simulink model "Electrical_System_2018b_obfs"  (R2019b)
settings: Solver=VariableStepAuto  StartTime=0.0  StopTime=5  RelTol=1e-3  AbsTol=1e-3  EnableMultiTasking=on
InitFcn:
  | Steady_State_Initialisation;
StopFcn:
  | %sscexplore(simlog);
  | %Logging
undefined symbols (not defined in the file): abrlhklxvp, aexgmhuedq, afmfmjnutg, afpphrjpnc, ahuxbyvruc, alarvljztt, amxnyqmnuw, aodrlwvqie, aolhmuplyq, aqpmguuqkg, auesgwirzl, aurophlnng, awamelrhru, ayfhvxflxn, azxkacuhqc, babszerikg, bawhdqanwq, bevoqecvei, bltjvqbchx, bmqsuewujl, bsmyqjfgnf, btvjbsmnve, bywgxqeadw, bziaduxaer, bzmcmdqocb, bzsvyvetat, ccsjnrbsih, cdvenygxwh, cedkrnslhx, cjheorclzs, cjrdshrtqx, ckhavyhcza, ckxewznhlz, cmrcgyiplk, conenicnws, cqkejbgjnn, csfnuwymhe, cunupkhwbh, cwzfvzuxxh, dcadmadufn, dcfponivnv, ddtrqjrhjn, dfhoxvkqas, dfrhtcwpne, dfvomcagjv, djijwylxea, dnmeqksrrm, dnzewbdkaa, dsqcykyxav, dtswwlttmm, ecumpidjtv, edegaywrct, ejjjsmnejc, eknqnehjdz, emvdetzouf, esxbqkbahr, etnkkbreiq, eunoiiiirw, ewewcuedir, fatkfxdhtc ... (+386)
libraries: fl_lib x802, ee_lib x362, fl_ps_legacy_lib x160, nesl_utility x85
(part 26 of 26)

== system Electrical_System_2018b_obfs/Redacted_1221/Redacted_7996/Redacted_7418/Redacted_4377/Redacted_6082/Redacted_3086/Redacted_7741 ==
  Redacted_4240 : fl_lib/Electrical/Electrical Elements/Open Circuit  v_specify=off  v_priority=None  v=ebhsjuvrvm V  v_nominal_specify=off  v_nominal_unit=V  v_nominal_value=uogdcjcffr
      settings: SourceProductName=Simscape  SourceProductBaseCode=SS
  Redacted_6054 : PMIOPort  Side=Left
  Redacted_5626 : PMIOPort  Port=2  Side=Left
  Redacted_6271 : PMIOPort  Port=3  Side=Left
  Redacted_2564 : PMIOPort  Port=4  Side=Right
  Redacted_7933 : PMIOPort  Port=5  Side=Right
  connections:
  Redacted_4240/LConn1 -- Redacted_5626/RConn1
  Redacted_2564/RConn1 -- Redacted_6054/RConn1
  Redacted_7933/RConn1 -- Redacted_6271/RConn1

== system Electrical_System_2018b_obfs/Redacted_1221/Redacted_7996/Redacted_7418/Redacted_4377/Redacted_6082/Redacted_3818/Neutral_Negative ==
  Open Circuit : fl_lib/Electrical/Electrical Elements/Open Circuit  v_specify=off  v_priority=None  v=0 V  v_nominal_specify=off  v_nominal_unit=V  v_nominal_value=1
      settings: SourceProductName=Simscape  SourceProductBaseCode=SS
  Redacted_558 : PMIOPort  Side=Left
  Redacted_9353 : PMIOPort  Port=2  Side=Left
  Redacted_2763 : PMIOPort  Port=3  Side=Left
  Redacted_5509 : PMIOPort  Port=4  Side=Right
  Redacted_3127 : PMIOPort  Port=5  Side=Right
  connections:
  Redacted_9353/RConn1 -- Redacted_5509/RConn1
  Open Circuit/LConn1 -- Redacted_558/RConn1
  Redacted_3127/RConn1 -- Redacted_2763/RConn1

== system Electrical_System_2018b_obfs/Redacted_1221/Redacted_7996/Redacted_7418/Redacted_4377/Redacted_6082/Redacted_3818/Positive_Neutral ==
  Open Circuit : fl_lib/Electrical/Electrical Elements/Open Circuit  v_specify=off  v_priority=None  v=0 V  v_nominal_specify=off  v_nominal_unit=V  v_nominal_value=1
      settings: SourceProductName=Simscape  SourceProductBaseCode=SS
  Redacted_558 : PMIOPort  Side=Left
  Redacted_9353 : PMIOPort  Port=2  Side=Left
  Redacted_2763 : PMIOPort  Port=3  Side=Left
  Redacted_5509 : PMIOPort  Port=4  Side=Right
  Redacted_3127 : PMIOPort  Port=5  Side=Right
  connections:
  Redacted_9353/RConn1 -- Redacted_3127/RConn1
  Redacted_5509/RConn1 -- Redacted_558/RConn1
  Open Circuit/LConn1 -- Redacted_2763/RConn1

== system Electrical_System_2018b_obfs/Redacted_1221/Redacted_7996/Redacted_7418/Redacted_4377/Redacted_6082/Redacted_3818/Redacted_7647 ==
  Redacted_9625 : fl_lib/Electrical/Electrical Elements/Open Circuit  v_specify=off  v_priority=None  v=ubfstcorvt V  v_nominal_specify=off  v_nominal_unit=V  v_nominal_value=abvsahtgbf
      settings: SourceProductName=Simscape  SourceProductBaseCode=SS
  Redacted_558 : PMIOPort  Side=Left
  Redacted_9353 : PMIOPort  Port=2  Side=Left
  Redacted_2763 : PMIOPort  Port=3  Side=Left
  Redacted_5509 : PMIOPort  Port=4  Side=Right
  Redacted_3127 : PMIOPort  Port=5  Side=Right
  connections:
  Redacted_3127/RConn1 -- Redacted_2763/RConn1
  Redacted_5509/RConn1 -- Redacted_558/RConn1
  Redacted_9625/LConn1 -- Redacted_9353/RConn1

== system Electrical_System_2018b_obfs/Redacted_1221/Redacted_7996/Redacted_7418/Redacted_4377/Redacted_6082/Redacted_4174/Neutral_Negative ==
  Open Circuit : fl_lib/Electrical/Electrical Elements/Open Circuit  v_specify=off  v_priority=None  v=0 V  v_nominal_specify=off  v_nominal_unit=V  v_nominal_value=1
      settings: SourceProductName=Simscape  SourceProductBaseCode=SS
  Redacted_9679 : PMIOPort  Side=Left
  Redacted_9878 : PMIOPort  Port=2  Side=Left
  Redacted_224 : PMIOPort  Port=3  Side=Left
  Redacted_5953 : PMIOPort  Port=4  Side=Right
  Redacted_7639 : PMIOPort  Port=5  Side=Right
  connections:
  Redacted_9878/RConn1 -- Redacted_5953/RConn1
  Open Circuit/LConn1 -- Redacted_9679/RConn1
  Redacted_7639/RConn1 -- Redacted_224/RConn1

== system Electrical_System_2018b_obfs/Redacted_1221/Redacted_7996/Redacted_7418/Redacted_4377/Redacted_6082/Redacted_4174/Positive_Neutral ==
  Open Circuit : fl_lib/Electrical/Electrical Elements/Open Circuit  v_specify=off  v_priority=None  v=0 V  v_nominal_specify=off  v_nominal_unit=V  v_nominal_value=1
      settings: SourceProductName=Simscape  SourceProductBaseCode=SS
  Redacted_9679 : PMIOPort  Side=Left
  Redacted_9878 : PMIOPort  Port=2  Side=Left
  Redacted_224 : PMIOPort  Port=3  Side=Left
  Redacted_5953 : PMIOPort  Port=4  Side=Right
  Redacted_7639 : PMIOPort  Port=5  Side=Right
  connections:
  Redacted_9878/RConn1 -- Redacted_7639/RConn1
  Redacted_5953/RConn1 -- Redacted_9679/RConn1
  Open Circuit/LConn1 -- Redacted_224/RConn1

== system Electrical_System_2018b_obfs/Redacted_1221/Redacted_7996/Redacted_7418/Redacted_4377/Redacted_6082/Redacted_4174/Redacted_8370 ==
  Redacted_7682 : fl_lib/Electrical/Electrical Elements/Open Circuit  v_specify=off  v_priority=None  v=krmygfnnpy V  v_nominal_specify=off  v_nominal_unit=V  v_nominal_value=lqikwmhyvq
      settings: SourceProductName=Simscape  SourceProductBaseCode=SS
  Redacted_9679 : PMIOPort  Side=Left
  Redacted_9878 : PMIOPort  Port=2  Side=Left
  Redacted_224 : PMIOPort  Port=3  Side=Left
  Redacted_5953 : PMIOPort  Port=4  Side=Right
  Redacted_7639 : PMIOPort  Port=5  Side=Right
  connections:
  Redacted_7639/RConn1 -- Redacted_224/RConn1
  Redacted_5953/RConn1 -- Redacted_9679/RConn1
  Redacted_7682/LConn1 -- Redacted_9878/RConn1

== system Electrical_System_2018b_obfs/Redacted_1221/Redacted_7996/Redacted_7418/Redacted_4377/Redacted_6082/Redacted_4278/Neutral_Negative ==
  Open Circuit : fl_lib/Electrical/Electrical Elements/Open Circuit  v_specify=off  v_priority=None  v=0 V  v_nominal_specify=off  v_nominal_unit=V  v_nominal_value=1
      settings: SourceProductName=Simscape  SourceProductBaseCode=SS
  Redacted_1495 : PMIOPort  Side=Left
  Redacted_2064 : PMIOPort  Port=2  Side=Left
  Redacted_9467 : PMIOPort  Port=3  Side=Left
  Redacted_1543 : PMIOPort  Port=4  Side=Right
  Redacted_9491 : PMIOPort  Port=5  Side=Right
  connections:
  Redacted_9491/RConn1 -- Redacted_9467/RConn1
  Open Circuit/LConn1 -- Redacted_1495/RConn1
  Redacted_2064/RConn1 -- Redacted_1543/RConn1

== system Electrical_System_2018b_obfs/Redacted_1221/Redacted_7996/Redacted_7418/Redacted_4377/Redacted_6082/Redacted_4278/Positive_Neutral ==
  Open Circuit : fl_lib/Electrical/Electrical Elements/Open Circuit  v_specify=off  v_priority=None  v=0 V  v_nominal_specify=off  v_nominal_unit=V  v_nominal_value=1
      settings: SourceProductName=Simscape  SourceProductBaseCode=SS
  Redacted_1495 : PMIOPort  Side=Left
  Redacted_2064 : PMIOPort  Port=2  Side=Left
  Redacted_9467 : PMIOPort  Port=3  Side=Left
  Redacted_1543 : PMIOPort  Port=4  Side=Right
  Redacted_9491 : PMIOPort  Port=5  Side=Right
  connections:
  Open Circuit/LConn1 -- Redacted_9467/RConn1
  Redacted_1543/RConn1 -- Redacted_1495/RConn1
  Redacted_2064/RConn1 -- Redacted_9491/RConn1

== system Electrical_System_2018b_obfs/Redacted_1221/Redacted_7996/Redacted_7418/Redacted_4377/Redacted_6082/Redacted_4278/Redacted_1592 ==
  Redacted_6518 : fl_lib/Electrical/Electrical Elements/Open Circuit  v_specify=off  v_priority=None  v=kniygukgpp V  v_nominal_specify=off  v_nominal_unit=V  v_nominal_value=dzkrotrooy
      settings: SourceProductName=Simscape  SourceProductBaseCode=SS
  Redacted_1495 : PMIOPort  Side=Left
  Redacted_2064 : PMIOPort  Port=2  Side=Left
  Redacted_9467 : PMIOPort  Port=3  Side=Left
  Redacted_1543 : PMIOPort  Port=4  Side=Right
  Redacted_9491 : PMIOPort  Port=5  Side=Right
  connections:
  Redacted_6518/LConn1 -- Redacted_2064/RConn1
  Redacted_1543/RConn1 -- Redacted_1495/RConn1
  Redacted_9491/RConn1 -- Redacted_9467/RConn1

== system Electrical_System_2018b_obfs/Redacted_1221/Redacted_7996/Redacted_7418/Redacted_4377/Redacted_6082/Redacted_4413/Neutral_Negative ==
  Open Circuit : fl_lib/Electrical/Electrical Elements/Open Circuit  v_specify=off  v_priority=None  v=0 V  v_nominal_specify=off  v_nominal_unit=V  v_nominal_value=1
      settings: SourceProductName=Simscape  SourceProductBaseCode=SS
  Redacted_9976 : PMIOPort  Side=Left
  Redacted_5180 : PMIOPort  Port=2  Side=Left
  Redacted_6712 : PMIOPort  Port=3  Side=Left
  Redacted_6595 : PMIOPort  Port=4  Side=Right
  Redacted_8408 : PMIOPort  Port=5  Side=Right
  connections:
  Redacted_8408/RConn1 -- Redacted_6712/RConn1
  Open Circuit/LConn1 -- Redacted_9976/RConn1
  Redacted_5180/RConn1 -- Redacted_6595/RConn1

== system Electrical_System_2018b_obfs/Redacted_1221/Redacted_7996/Redacted_7418/Redacted_4377/Redacted_6082/Redacted_4413/Positive_Neutral ==
  Open Circuit : fl_lib/Electrical/Electrical Elements/Open Circuit  v_specify=off  v_priority=None  v=0 V  v_nominal_specify=off  v_nominal_unit=V  v_nominal_value=1
      settings: SourceProductName=Simscape  SourceProductBaseCode=SS
  Redacted_9976 : PMIOPort  Side=Left
  Redacted_5180 : PMIOPort  Port=2  Side=Left
  Redacted_6712 : PMIOPort  Port=3  Side=Left
  Redacted_6595 : PMIOPort  Port=4  Side=Right
  Redacted_8408 : PMIOPort  Port=5  Side=Right
  connections:
  Open Circuit/LConn1 -- Redacted_6712/RConn1
  Redacted_6595/RConn1 -- Redacted_9976/RConn1
  Redacted_5180/RConn1 -- Redacted_8408/RConn1

== system Electrical_System_2018b_obfs/Redacted_1221/Redacted_7996/Redacted_7418/Redacted_4377/Redacted_6082/Redacted_4413/Redacted_6190 ==
  Redacted_6825 : fl_lib/Electrical/Electrical Elements/Open Circuit  v_specify=off  v_priority=None  v=nafaxblafc V  v_nominal_specify=off  v_nominal_unit=V  v_nominal_value=uctqgjleyg
      settings: SourceProductName=Simscape  SourceProductBaseCode=SS
  Redacted_9976 : PMIOPort  Side=Left
  Redacted_5180 : PMIOPort  Port=2  Side=Left
  Redacted_6712 : PMIOPort  Port=3  Side=Left
  Redacted_6595 : PMIOPort  Port=4  Side=Right
  Redacted_8408 : PMIOPort  Port=5  Side=Right
  connections:
  Redacted_6825/LConn1 -- Redacted_5180/RConn1
  Redacted_6595/RConn1 -- Redacted_9976/RConn1
  Redacted_8408/RConn1 -- Redacted_6712/RConn1

== system Electrical_System_2018b_obfs/Redacted_1221/Redacted_7996/Redacted_7418/Redacted_4377/Redacted_6082/Redacted_5550/Neutral_Negative ==
  Open Circuit : fl_lib/Electrical/Electrical Elements/Open Circuit  v_specify=off  v_priority=None  v=0 V  v_nominal_specify=off  v_nominal_unit=V  v_nominal_value=1
      settings: SourceProductName=Simscape  SourceProductBaseCode=SS
  Redacted_6826 : PMIOPort  Side=Left
  Redacted_51 : PMIOPort  Port=2  Side=Left
  Redacted_9515 : PMIOPort  Port=3  Side=Left
  Redacted_375 : PMIOPort  Port=4  Side=Right
  Redacted_6304 : PMIOPort  Port=5  Side=Right
  connections:
  Redacted_6304/RConn1 -- Redacted_9515/RConn1
  Open Circuit/LConn1 -- Redacted_6826/RConn1
  Redacted_51/RConn1 -- Redacted_375/RConn1

== system Electrical_System_2018b_obfs/Redacted_1221/Redacted_7996/Redacted_7418/Redacted_4377/Redacted_6082/Redacted_5550/Positive_Neutral ==
  Open Circuit : fl_lib/Electrical/Electrical Elements/Open Circuit  v_specify=off  v_priority=None  v=0 V  v_nominal_specify=off  v_nominal_unit=V  v_nominal_value=1
      settings: SourceProductName=Simscape  SourceProductBaseCode=SS
  Redacted_6826 : PMIOPort  Side=Left
  Redacted_51 : PMIOPort  Port=2  Side=Left
  Redacted_9515 : PMIOPort  Port=3  Side=Left
  Redacted_375 : PMIOPort  Port=4  Side=Right
  Redacted_6304 : PMIOPort  Port=5  Side=Right
  connections:
  Open Circuit/LConn1 -- Redacted_9515/RConn1
  Redacted_375/RConn1 -- Redacted_6826/RConn1
  Redacted_51/RConn1 -- Redacted_6304/RConn1

== system Electrical_System_2018b_obfs/Redacted_1221/Redacted_7996/Redacted_7418/Redacted_4377/Redacted_6082/Redacted_5550/Redacted_2952 ==
  Redacted_9904 : fl_lib/Electrical/Electrical Elements/Open Circuit  v_specify=off  v_priority=None  v=cbwtykvznf V  v_nominal_specify=off  v_nominal_unit=V  v_nominal_value=bbwdbtprkb
      settings: SourceProductName=Simscape  SourceProductBaseCode=SS
  Redacted_6826 : PMIOPort  Side=Left
  Redacted_51 : PMIOPort  Port=2  Side=Left
  Redacted_9515 : PMIOPort  Port=3  Side=Left
  Redacted_375 : PMIOPort  Port=4  Side=Right
  Redacted_6304 : PMIOPort  Port=5  Side=Right
  connections:
  Redacted_9904/LConn1 -- Redacted_51/RConn1
  Redacted_375/RConn1 -- Redacted_6826/RConn1
  Redacted_6304/RConn1 -- Redacted_9515/RConn1

== system Electrical_System_2018b_obfs/Redacted_1221/Redacted_7996/Redacted_7418/Redacted_4377/Redacted_6082/Redacted_5713/Neutral_Negative ==
  Open Circuit : fl_lib/Electrical/Electrical Elements/Open Circuit  v_specify=off  v_priority=None  v=0 V  v_nominal_specify=off  v_nominal_unit=V  v_nominal_value=1
      settings: SourceProductName=Simscape  SourceProductBaseCode=SS
  Redacted_6138 : PMIOPort  Side=Left
  Redacted_1431 : PMIOPort  Port=2  Side=Left
  Redacted_7946 : PMIOPort  Port=3  Side=Left
  Redacted_819 : PMIOPort  Port=4  Side=Right
  Redacted_4816 : PMIOPort  Port=5  Side=Right
  connections:
  Redacted_4816/RConn1 -- Redacted_7946/RConn1
  Open Circuit/LConn1 -- Redacted_6138/RConn1
  Redacted_1431/RConn1 -- Redacted_819/RConn1

== system Electrical_System_2018b_obfs/Redacted_1221/Redacted_7996/Redacted_7418/Redacted_4377/Redacted_6082/Redacted_5713/Positive_Neutral ==
  Open Circuit : fl_lib/Electrical/Electrical Elements/Open Circuit  v_specify=off  v_priority=None  v=0 V  v_nominal_specify=off  v_nominal_unit=V  v_nominal_value=1
      settings: SourceProductName=Simscape  SourceProductBaseCode=SS
  Redacted_6138 : PMIOPort  Side=Left
  Redacted_1431 : PMIOPort  Port=2  Side=Left
  Redacted_7946 : PMIOPort  Port=3  Side=Left
  Redacted_819 : PMIOPort  Port=4  Side=Right
  Redacted_4816 : PMIOPort  Port=5  Side=Right
  connections:
  Open Circuit/LConn1 -- Redacted_7946/RConn1
  Redacted_819/RConn1 -- Redacted_6138/RConn1
  Redacted_1431/RConn1 -- Redacted_4816/RConn1

== system Electrical_System_2018b_obfs/Redacted_1221/Redacted_7996/Redacted_7418/Redacted_4377/Redacted_6082/Redacted_5713/Redacted_1184 ==
  Redacted_2299 : fl_lib/Electrical/Electrical Elements/Open Circuit  v_specify=off  v_priority=None  v=tqpmitufxi V  v_nominal_specify=off  v_nominal_unit=V  v_nominal_value=nizvadugds
      settings: SourceProductName=Simscape  SourceProductBaseCode=SS
  Redacted_6138 : PMIOPort  Side=Left
  Redacted_1431 : PMIOPort  Port=2  Side=Left
  Redacted_7946 : PMIOPort  Port=3  Side=Left
  Redacted_819 : PMIOPort  Port=4  Side=Right
  Redacted_4816 : PMIOPort  Port=5  Side=Right
  connections:
  Redacted_2299/LConn1 -- Redacted_1431/RConn1
  Redacted_819/RConn1 -- Redacted_6138/RConn1
  Redacted_4816/RConn1 -- Redacted_7946/RConn1

== system Electrical_System_2018b_obfs/Redacted_1221/Redacted_7996/Redacted_7418/Redacted_4377/Redacted_6082/Redacted_5976/Neutral_Negative ==
  Open Circuit : fl_lib/Electrical/Electrical Elements/Open Circuit  v_specify=off  v_priority=None  v=0 V  v_nominal_specify=off  v_nominal_unit=V  v_nominal_value=1
      settings: SourceProductName=Simscape  SourceProductBaseCode=SS
  Redacted_9241 : PMIOPort  Side=Left
  Redacted_5276 : PMIOPort  Port=2  Side=Left
  Redacted_2400 : PMIOPort  Port=3  Side=Left
  Redacted_5406 : PMIOPort  Port=4  Side=Right
  Redacted_1074 : PMIOPort  Port=5  Side=Right
  connections:
  Redacted_5276/RConn1 -- Redacted_5406/RConn1
  Open Circuit/LConn1 -- Redacted_9241/RConn1
  Redacted_1074/RConn1 -- Redacted_2400/RConn1

== system Electrical_System_2018b_obfs/Redacted_1221/Redacted_7996/Redacted_7418/Redacted_4377/Redacted_6082/Redacted_5976/Positive_Neutral ==
  Open Circuit : fl_lib/Electrical/Electrical Elements/Open Circuit  v_specify=off  v_priority=None  v=0 V  v_nominal_specify=off  v_nominal_unit=V  v_nominal_value=1
      settings: SourceProductName=Simscape  SourceProductBaseCode=SS
  Redacted_9241 : PMIOPort  Side=Left
  Redacted_5276 : PMIOPort  Port=2  Side=Left
  Redacted_2400 : PMIOPort  Port=3  Side=Left
  Redacted_5406 : PMIOPort  Port=4  Side=Right
  Redacted_1074 : PMIOPort  Port=5  Side=Right
  connections:
  Redacted_5276/RConn1 -- Redacted_1074/RConn1
  Redacted_5406/RConn1 -- Redacted_9241/RConn1
  Open Circuit/LConn1 -- Redacted_2400/RConn1

== system Electrical_System_2018b_obfs/Redacted_1221/Redacted_7996/Redacted_7418/Redacted_4377/Redacted_6082/Redacted_5976/Redacted_5620 ==
  Redacted_9178 : fl_lib/Electrical/Electrical Elements/Open Circuit  v_specify=off  v_priority=None  v=jhtpowznxh V  v_nominal_specify=off  v_nominal_unit=V  v_nominal_value=mubuuhzqmu
      settings: SourceProductName=Simscape  SourceProductBaseCode=SS
  Redacted_9241 : PMIOPort  Side=Left
  Redacted_5276 : PMIOPort  Port=2  Side=Left
  Redacted_2400 : PMIOPort  Port=3  Side=Left
  Redacted_5406 : PMIOPort  Port=4  Side=Right
  Redacted_1074 : PMIOPort  Port=5  Side=Right
  connections:
  Redacted_1074/RConn1 -- Redacted_2400/RConn1
  Redacted_5406/RConn1 -- Redacted_9241/RConn1
  Redacted_9178/LConn1 -- Redacted_5276/RConn1

== system Electrical_System_2018b_obfs/Redacted_1221/Redacted_7996/Redacted_7418/Redacted_4377/Redacted_6082/Redacted_6424/Neutral_Negative ==
  Open Circuit : fl_lib/Electrical/Electrical Elements/Open Circuit  v_specify=off  v_priority=None  v=0 V  v_nominal_specify=off  v_nominal_unit=V  v_nominal_value=1
      settings: SourceProductName=Simscape  SourceProductBaseCode=SS
  Redacted_4582 : PMIOPort  Side=Left
  Redacted_1544 : PMIOPort  Port=2  Side=Left
  Redacted_1581 : PMIOPort  Port=3  Side=Left
  Redacted_1961 : PMIOPort  Port=4  Side=Right
  Redacted_7479 : PMIOPort  Port=5  Side=Right
  connections:
  Redacted_7479/RConn1 -- Redacted_1581/RConn1
  Open Circuit/LConn1 -- Redacted_4582/RConn1
  Redacted_1544/RConn1 -- Redacted_1961/RConn1

== system Electrical_System_2018b_obfs/Redacted_1221/Redacted_7996/Redacted_7418/Redacted_4377/Redacted_6082/Redacted_6424/Positive_Neutral ==
  Open Circuit : fl_lib/Electrical/Electrical Elements/Open Circuit  v_specify=off  v_priority=None  v=0 V  v_nominal_specify=off  v_nominal_unit=V  v_nominal_value=1
      settings: SourceProductName=Simscape  SourceProductBaseCode=SS
  Redacted_4582 : PMIOPort  Side=Left
  Redacted_1544 : PMIOPort  Port=2  Side=Left
  Redacted_1581 : PMIOPort  Port=3  Side=Left
  Redacted_1961 : PMIOPort  Port=4  Side=Right
  Redacted_7479 : PMIOPort  Port=5  Side=Right
  connections:
  Open Circuit/LConn1 -- Redacted_1581/RConn1
  Redacted_1961/RConn1 -- Redacted_4582/RConn1
  Redacted_1544/RConn1 -- Redacted_7479/RConn1

== system Electrical_System_2018b_obfs/Redacted_1221/Redacted_7996/Redacted_7418/Redacted_4377/Redacted_6082/Redacted_6424/Redacted_7805 ==
  Redacted_3936 : fl_lib/Electrical/Electrical Elements/Open Circuit  v_specify=off  v_priority=None  v=fjoxglgvhp V  v_nominal_specify=off  v_nominal_unit=V  v_nominal_value=omyuclhrqc
      settings: SourceProductName=Simscape  SourceProductBaseCode=SS
  Redacted_4582 : PMIOPort  Side=Left
  Redacted_1544 : PMIOPort  Port=2  Side=Left
  Redacted_1581 : PMIOPort  Port=3  Side=Left
  Redacted_1961 : PMIOPort  Port=4  Side=Right
  Redacted_7479 : PMIOPort  Port=5  Side=Right
  connections:
  Redacted_3936/LConn1 -- Redacted_1544/RConn1
  Redacted_1961/RConn1 -- Redacted_4582/RConn1
  Redacted_7479/RConn1 -- Redacted_1581/RConn1

== system Electrical_System_2018b_obfs/Redacted_1221/Redacted_7996/Redacted_7418/Redacted_4377/Redacted_6082/Redacted_7051/Neutral_Negative ==
  Open Circuit : fl_lib/Electrical/Electrical Elements/Open Circuit  v_specify=off  v_priority=None  v=0 V  v_nominal_specify=off  v_nominal_unit=V  v_nominal_value=1
      settings: SourceProductName=Simscape  SourceProductBaseCode=SS
  Redacted_2697 : PMIOPort  Side=Left
  Redacted_1518 : PMIOPort  Port=2  Side=Left
  Redacted_2395 : PMIOPort  Port=3  Side=Left
  Redacted_3537 : PMIOPort  Port=4  Side=Right
  Redacted_8383 : PMIOPort  Port=5  Side=Right
  connections:
  Redacted_1518/RConn1 -- Redacted_3537/RConn1
  Open Circuit/LConn1 -- Redacted_2697/RConn1
  Redacted_8383/RConn1 -- Redacted_2395/RConn1

== system Electrical_System_2018b_obfs/Redacted_1221/Redacted_7996/Redacted_7418/Redacted_4377/Redacted_6082/Redacted_7051/Positive_Neutral ==
  Open Circuit : fl_lib/Electrical/Electrical Elements/Open Circuit  v_specify=off  v_priority=None  v=0 V  v_nominal_specify=off  v_nominal_unit=V  v_nominal_value=1
      settings: SourceProductName=Simscape  SourceProductBaseCode=SS
  Redacted_2697 : PMIOPort  Side=Left
  Redacted_1518 : PMIOPort  Port=2  Side=Left
  Redacted_2395 : PMIOPort  Port=3  Side=Left
  Redacted_3537 : PMIOPort  Port=4  Side=Right
  Redacted_8383 : PMIOPort  Port=5  Side=Right
  connections:
  Redacted_1518/RConn1 -- Redacted_8383/RConn1
  Redacted_3537/RConn1 -- Redacted_2697/RConn1
  Open Circuit/LConn1 -- Redacted_2395/RConn1

== system Electrical_System_2018b_obfs/Redacted_1221/Redacted_7996/Redacted_7418/Redacted_4377/Redacted_6082/Redacted_7051/Redacted_1021 ==
  Redacted_3666 : fl_lib/Electrical/Electrical Elements/Open Circuit  v_specify=off  v_priority=None  v=jitpzdpdri V  v_nominal_specify=off  v_nominal_unit=V  v_nominal_value=zhywmqlonq
      settings: SourceProductName=Simscape  SourceProductBaseCode=SS
  Redacted_2697 : PMIOPort  Side=Left
  Redacted_1518 : PMIOPort  Port=2  Side=Left
  Redacted_2395 : PMIOPort  Port=3  Side=Left
  Redacted_3537 : PMIOPort  Port=4  Side=Right
  Redacted_8383 : PMIOPort  Port=5  Side=Right
  connections:
  Redacted_8383/RConn1 -- Redacted_2395/RConn1
  Redacted_3537/RConn1 -- Redacted_2697/RConn1
  Redacted_3666/LConn1 -- Redacted_1518/RConn1

== system Electrical_System_2018b_obfs/Redacted_1221/Redacted_7996/Redacted_7418/Redacted_4377/Redacted_6082/Redacted_7884/Neutral_Negative ==
  Open Circuit : fl_lib/Electrical/Electrical Elements/Open Circuit  v_specify=off  v_priority=None  v=0 V  v_nominal_specify=off  v_nominal_unit=V  v_nominal_value=1
      settings: SourceProductName=Simscape  SourceProductBaseCode=SS
  Redacted_6224 : PMIOPort  Side=Left
  Redacted_4321 : PMIOPort  Port=2  Side=Left
  Redacted_2243 : PMIOPort  Port=3  Side=Left
  Redacted_707 : PMIOPort  Port=4  Side=Right
  Redacted_8636 : PMIOPort  Port=5  Side=Right
  connections:
  Redacted_4321/RConn1 -- Redacted_707/RConn1
  Open Circuit/LConn1 -- Redacted_6224/RConn1
  Redacted_8636/RConn1 -- Redacted_2243/RConn1

== system Electrical_System_2018b_obfs/Redacted_1221/Redacted_7996/Redacted_7418/Redacted_4377/Redacted_6082/Redacted_7884/Positive_Neutral ==
  Open Circuit : fl_lib/Electrical/Electrical Elements/Open Circuit  v_specify=off  v_priority=None  v=0 V  v_nominal_specify=off  v_nominal_unit=V  v_nominal_value=1
      settings: SourceProductName=Simscape  SourceProductBaseCode=SS
  Redacted_6224 : PMIOPort  Side=Left
  Redacted_4321 : PMIOPort  Port=2  Side=Left
  Redacted_2243 : PMIOPort  Port=3  Side=Left
  Redacted_707 : PMIOPort  Port=4  Side=Right
  Redacted_8636 : PMIOPort  Port=5  Side=Right
  connections:
  Redacted_4321/RConn1 -- Redacted_8636/RConn1
  Redacted_707/RConn1 -- Redacted_6224/RConn1
  Open Circuit/LConn1 -- Redacted_2243/RConn1

== system Electrical_System_2018b_obfs/Redacted_1221/Redacted_7996/Redacted_7418/Redacted_4377/Redacted_6082/Redacted_7884/Redacted_81 ==
  Redacted_8822 : fl_lib/Electrical/Electrical Elements/Open Circuit  v_specify=off  v_priority=None  v=nrbmgkomdb V  v_nominal_specify=off  v_nominal_unit=V  v_nominal_value=chrfcotgkg
      settings: SourceProductName=Simscape  SourceProductBaseCode=SS
  Redacted_6224 : PMIOPort  Side=Left
  Redacted_4321 : PMIOPort  Port=2  Side=Left
  Redacted_2243 : PMIOPort  Port=3  Side=Left
  Redacted_707 : PMIOPort  Port=4  Side=Right
  Redacted_8636 : PMIOPort  Port=5  Side=Right
  connections:
  Redacted_8636/RConn1 -- Redacted_2243/RConn1
  Redacted_707/RConn1 -- Redacted_6224/RConn1
  Redacted_8822/LConn1 -- Redacted_4321/RConn1

== system Electrical_System_2018b_obfs/Redacted_1221/Redacted_7996/Redacted_7418/Redacted_4377/Redacted_6082/Redacted_8502/Neutral_Negative ==
  Open Circuit : fl_lib/Electrical/Electrical Elements/Open Circuit  v_specify=off  v_priority=None  v=0 V  v_nominal_specify=off  v_nominal_unit=V  v_nominal_value=1
      settings: SourceProductName=Simscape  SourceProductBaseCode=SS
  Redacted_389 : PMIOPort  Side=Left
  Redacted_6488 : PMIOPort  Port=2  Side=Left
  Redacted_5156 : PMIOPort  Port=3  Side=Left
  Redacted_180 : PMIOPort  Port=4  Side=Right
  Redacted_7018 : PMIOPort  Port=5  Side=Right
  connections:
  Redacted_6488/RConn1 -- Redacted_180/RConn1
  Open Circuit/LConn1 -- Redacted_389/RConn1
  Redacted_7018/RConn1 -- Redacted_5156/RConn1

== system Electrical_System_2018b_obfs/Redacted_1221/Redacted_7996/Redacted_7418/Redacted_4377/Redacted_6082/Redacted_8502/Positive_Neutral ==
  Open Circuit : fl_lib/Electrical/Electrical Elements/Open Circuit  v_specify=off  v_priority=None  v=0 V  v_nominal_specify=off  v_nominal_unit=V  v_nominal_value=1
      settings: SourceProductName=Simscape  SourceProductBaseCode=SS
  Redacted_389 : PMIOPort  Side=Left
  Redacted_6488 : PMIOPort  Port=2  Side=Left
  Redacted_5156 : PMIOPort  Port=3  Side=Left
  Redacted_180 : PMIOPort  Port=4  Side=Right
  Redacted_7018 : PMIOPort  Port=5  Side=Right
  connections:
  Redacted_6488/RConn1 -- Redacted_7018/RConn1
  Redacted_180/RConn1 -- Redacted_389/RConn1
  Open Circuit/LConn1 -- Redacted_5156/RConn1

== system Electrical_System_2018b_obfs/Redacted_1221/Redacted_7996/Redacted_7418/Redacted_4377/Redacted_6082/Redacted_8502/Redacted_4068 ==
  Redacted_9772 : fl_lib/Electrical/Electrical Elements/Open Circuit  v_specify=off  v_priority=None  v=truhycjrml V  v_nominal_specify=off  v_nominal_unit=V  v_nominal_value=fuzhyyoiey
      settings: SourceProductName=Simscape  SourceProductBaseCode=SS
  Redacted_389 : PMIOPort  Side=Left
  Redacted_6488 : PMIOPort  Port=2  Side=Left
  Redacted_5156 : PMIOPort  Port=3  Side=Left
  Redacted_180 : PMIOPort  Port=4  Side=Right
  Redacted_7018 : PMIOPort  Port=5  Side=Right
  connections:
  Redacted_7018/RConn1 -- Redacted_5156/RConn1
  Redacted_180/RConn1 -- Redacted_389/RConn1
  Redacted_9772/LConn1 -- Redacted_6488/RConn1

== system Electrical_System_2018b_obfs/Redacted_1221/Redacted_7996/Redacted_7418/Redacted_4377/Redacted_6082/Redacted_9034/Neutral_Negative ==
  Open Circuit : fl_lib/Electrical/Electrical Elements/Open Circuit  v_specify=off  v_priority=None  v=0 V  v_nominal_specify=off  v_nominal_unit=V  v_nominal_value=1
      settings: SourceProductName=Simscape  SourceProductBaseCode=SS
  Redacted_4887 : PMIOPort  Side=Left
  Redacted_5529 : PMIOPort  Port=2  Side=Left
  Redacted_4069 : PMIOPort  Port=3  Side=Left
  Redacted_1826 : PMIOPort  Port=4  Side=Right
  Redacted_1222 : PMIOPort  Port=5  Side=Right
  connections:
  Redacted_1222/RConn1 -- Redacted_4069/RConn1
  Open Circuit/LConn1 -- Redacted_4887/RConn1
  Redacted_5529/RConn1 -- Redacted_1826/RConn1

== system Electrical_System_2018b_obfs/Redacted_1221/Redacted_7996/Redacted_7418/Redacted_4377/Redacted_6082/Redacted_9034/Positive_Neutral ==
  Open Circuit : fl_lib/Electrical/Electrical Elements/Open Circuit  v_specify=off  v_priority=None  v=0 V  v_nominal_specify=off  v_nominal_unit=V  v_nominal_value=1
      settings: SourceProductName=Simscape  SourceProductBaseCode=SS
  Redacted_4887 : PMIOPort  Side=Left
  Redacted_5529 : PMIOPort  Port=2  Side=Left
  Redacted_4069 : PMIOPort  Port=3  Side=Left
  Redacted_1826 : PMIOPort  Port=4  Side=Right
  Redacted_1222 : PMIOPort  Port=5  Side=Right
  connections:
  Open Circuit/LConn1 -- Redacted_4069/RConn1
  Redacted_1826/RConn1 -- Redacted_4887/RConn1
  Redacted_5529/RConn1 -- Redacted_1222/RConn1

== system Electrical_System_2018b_obfs/Redacted_1221/Redacted_7996/Redacted_7418/Redacted_4377/Redacted_6082/Redacted_9034/Redacted_4182 ==
  Redacted_1436 : fl_lib/Electrical/Electrical Elements/Open Circuit  v_specify=off  v_priority=None  v=zzrofiuybt V  v_nominal_specify=off  v_nominal_unit=V  v_nominal_value=ignlzzzuid
      settings: SourceProductName=Simscape  SourceProductBaseCode=SS
  Redacted_4887 : PMIOPort  Side=Left
  Redacted_5529 : PMIOPort  Port=2  Side=Left
  Redacted_4069 : PMIOPort  Port=3  Side=Left
  Redacted_1826 : PMIOPort  Port=4  Side=Right
  Redacted_1222 : PMIOPort  Port=5  Side=Right
  connections:
  Redacted_1436/LConn1 -- Redacted_5529/RConn1
  Redacted_1826/RConn1 -- Redacted_4887/RConn1
  Redacted_1222/RConn1 -- Redacted_4069/RConn1

== system Electrical_System_2018b_obfs/Redacted_1221/Redacted_7996/Redacted_7418/Redacted_4377/Redacted_6082/Redacted_9572/Neutral_Negative ==
  Open Circuit : fl_lib/Electrical/Electrical Elements/Open Circuit  v_specify=off  v_priority=None  v=0 V  v_nominal_specify=off  v_nominal_unit=V  v_nominal_value=1
      settings: SourceProductName=Simscape  SourceProductBaseCode=SS
  Redacted_435 : PMIOPort  Side=Left
  Redacted_1376 : PMIOPort  Port=2  Side=Left
  Redacted_8237 : PMIOPort  Port=3  Side=Left
  Redacted_4941 : PMIOPort  Port=4  Side=Right
  Redacted_729 : PMIOPort  Port=5  Side=Right
  connections:
  Redacted_1376/RConn1 -- Redacted_4941/RConn1
  Open Circuit/LConn1 -- Redacted_435/RConn1
  Redacted_729/RConn1 -- Redacted_8237/RConn1

== system Electrical_System_2018b_obfs/Redacted_1221/Redacted_7996/Redacted_7418/Redacted_4377/Redacted_6082/Redacted_9572/Positive_Neutral ==
  Open Circuit : fl_lib/Electrical/Electrical Elements/Open Circuit  v_specify=off  v_priority=None  v=0 V  v_nominal_specify=off  v_nominal_unit=V  v_nominal_value=1
      settings: SourceProductName=Simscape  SourceProductBaseCode=SS
  Redacted_435 : PMIOPort  Side=Left
  Redacted_1376 : PMIOPort  Port=2  Side=Left
  Redacted_8237 : PMIOPort  Port=3  Side=Left
  Redacted_4941 : PMIOPort  Port=4  Side=Right
  Redacted_729 : PMIOPort  Port=5  Side=Right
  connections:
  Redacted_1376/RConn1 -- Redacted_729/RConn1
  Redacted_4941/RConn1 -- Redacted_435/RConn1
  Open Circuit/LConn1 -- Redacted_8237/RConn1

== system Electrical_System_2018b_obfs/Redacted_1221/Redacted_7996/Redacted_7418/Redacted_4377/Redacted_6082/Redacted_9572/Redacted_3288 ==
  Redacted_4505 : fl_lib/Electrical/Electrical Elements/Open Circuit  v_specify=off  v_priority=None  v=bjybeoqvmc V  v_nominal_specify=off  v_nominal_unit=V  v_nominal_value=ldxcbaigcw
      settings: SourceProductName=Simscape  SourceProductBaseCode=SS
  Redacted_435 : PMIOPort  Side=Left
  Redacted_1376 : PMIOPort  Port=2  Side=Left
  Redacted_8237 : PMIOPort  Port=3  Side=Left
  Redacted_4941 : PMIOPort  Port=4  Side=Right
  Redacted_729 : PMIOPort  Port=5  Side=Right
  connections:
  Redacted_729/RConn1 -- Redacted_8237/RConn1
  Redacted_4941/RConn1 -- Redacted_435/RConn1
  Redacted_4505/LConn1 -- Redacted_1376/RConn1

== system Electrical_System_2018b_obfs/Redacted_1221/Redacted_7996/Redacted_7418/Redacted_4377/Redacted_6082/Redacted_980/Neutral_Negative ==
  Open Circuit : fl_lib/Electrical/Electrical Elements/Open Circuit  v_specify=off  v_priority=None  v=0 V  v_nominal_specify=off  v_nominal_unit=V  v_nominal_value=1
      settings: SourceProductName=Simscape  SourceProductBaseCode=SS
  Redacted_3281 : PMIOPort  Side=Left
  Redacted_9175 : PMIOPort  Port=2  Side=Left
  Redacted_1087 : PMIOPort  Port=3  Side=Left
  Redacted_2672 : PMIOPort  Port=4  Side=Right
  Redacted_3599 : PMIOPort  Port=5  Side=Right
  connections:
  Redacted_3599/RConn1 -- Redacted_1087/RConn1
  Open Circuit/LConn1 -- Redacted_3281/RConn1
  Redacted_9175/RConn1 -- Redacted_2672/RConn1

== system Electrical_System_2018b_obfs/Redacted_1221/Redacted_7996/Redacted_7418/Redacted_4377/Redacted_6082/Redacted_980/Positive_Neutral ==
  Open Circuit : fl_lib/Electrical/Electrical Elements/Open Circuit  v_specify=off  v_priority=None  v=0 V  v_nominal_specify=off  v_nominal_unit=V  v_nominal_value=1
      settings: SourceProductName=Simscape  SourceProductBaseCode=SS
  Redacted_3281 : PMIOPort  Side=Left
  Redacted_9175 : PMIOPort  Port=2  Side=Left
  Redacted_1087 : PMIOPort  Port=3  Side=Left
  Redacted_2672 : PMIOPort  Port=4  Side=Right
  Redacted_3599 : PMIOPort  Port=5  Side=Right
  connections:
  Open Circuit/LConn1 -- Redacted_1087/RConn1
  Redacted_2672/RConn1 -- Redacted_3281/RConn1
  Redacted_9175/RConn1 -- Redacted_3599/RConn1

== system Electrical_System_2018b_obfs/Redacted_1221/Redacted_7996/Redacted_7418/Redacted_4377/Redacted_6082/Redacted_980/Redacted_8833 ==
  Redacted_4926 : fl_lib/Electrical/Electrical Elements/Open Circuit  v_specify=off  v_priority=None  v=pdiyatassn V  v_nominal_specify=off  v_nominal_unit=V  v_nominal_value=uflvhyhiqw
      settings: SourceProductName=Simscape  SourceProductBaseCode=SS
  Redacted_3281 : PMIOPort  Side=Left
  Redacted_9175 : PMIOPort  Port=2  Side=Left
  Redacted_1087 : PMIOPort  Port=3  Side=Left
  Redacted_2672 : PMIOPort  Port=4  Side=Right
  Redacted_3599 : PMIOPort  Port=5  Side=Right
  connections:
  Redacted_4926/LConn1 -- Redacted_9175/RConn1
  Redacted_2672/RConn1 -- Redacted_3281/RConn1
  Redacted_3599/RConn1 -- Redacted_1087/RConn1

== system Electrical_System_2018b_obfs/Redacted_1221/Redacted_7996/Redacted_9242/Redacted_38/Redacted_8107/Redacted_3070/Neutral_Negative ==
  Open Circuit : fl_lib/Electrical/Electrical Elements/Open Circuit  v_specify=off  v_priority=None  v=0 V  v_nominal_specify=off  v_nominal_unit=V  v_nominal_value=1
      settings: SourceProductName=Simscape  SourceProductBaseCode=SS
  Redacted_9800 : PMIOPort  Side=Left
  Redacted_6600 : PMIOPort  Port=2  Side=Left
  Redacted_5239 : PMIOPort  Port=3  Side=Left
  Redacted_3081 : PMIOPort  Port=4  Side=Right
  Redacted_7642 : PMIOPort  Port=5  Side=Right
  connections:
  Redacted_6600/RConn1 -- Redacted_3081/RConn1
  Open Circuit/LConn1 -- Redacted_9800/RConn1
  Redacted_7642/RConn1 -- Redacted_5239/RConn1

== system Electrical_System_2018b_obfs/Redacted_1221/Redacted_7996/Redacted_9242/Redacted_38/Redacted_8107/Redacted_3070/Positive_Neutral ==
  Open Circuit : fl_lib/Electrical/Electrical Elements/Open Circuit  v_specify=off  v_priority=None  v=0 V  v_nominal_specify=off  v_nominal_unit=V  v_nominal_value=1
      settings: SourceProductName=Simscape  SourceProductBaseCode=SS
  Redacted_9800 : PMIOPort  Side=Left
  Redacted_6600 : PMIOPort  Port=2  Side=Left
  Redacted_5239 : PMIOPort  Port=3  Side=Left
  Redacted_3081 : PMIOPort  Port=4  Side=Right
  Redacted_7642 : PMIOPort  Port=5  Side=Right
  connections:
  Redacted_6600/RConn1 -- Redacted_7642/RConn1
  Redacted_3081/RConn1 -- Redacted_9800/RConn1
  Open Circuit/LConn1 -- Redacted_5239/RConn1

== system Electrical_System_2018b_obfs/Redacted_1221/Redacted_7996/Redacted_9242/Redacted_38/Redacted_8107/Redacted_3070/Redacted_6581 ==
  Redacted_9951 : fl_lib/Electrical/Electrical Elements/Open Circuit  v_specify=off  v_priority=None  v=kbecunztrl V  v_nominal_specify=off  v_nominal_unit=V  v_nominal_value=jkubweymaj
      settings: SourceProductName=Simscape  SourceProductBaseCode=SS
  Redacted_9800 : PMIOPort  Side=Left
  Redacted_6600 : PMIOPort  Port=2  Side=Left
  Redacted_5239 : PMIOPort  Port=3  Side=Left
  Redacted_3081 : PMIOPort  Port=4  Side=Right
  Redacted_7642 : PMIOPort  Port=5  Side=Right
  connections:
  Redacted_7642/RConn1 -- Redacted_5239/RConn1
  Redacted_3081/RConn1 -- Redacted_9800/RConn1
  Redacted_9951/LConn1 -- Redacted_6600/RConn1

== system Electrical_System_2018b_obfs/Redacted_1221/Redacted_7996/Redacted_9242/Redacted_38/Redacted_8107/Redacted_8444/Neutral_Negative ==
  Open Circuit : fl_lib/Electrical/Electrical Elements/Open Circuit  v_specify=off  v_priority=None  v=0 V  v_nominal_specify=off  v_nominal_unit=V  v_nominal_value=1
      settings: SourceProductName=Simscape  SourceProductBaseCode=SS
  Redacted_8974 : PMIOPort  Side=Left
  Redacted_9727 : PMIOPort  Port=2  Side=Left
  Redacted_5818 : PMIOPort  Port=3  Side=Left
  Redacted_9930 : PMIOPort  Port=4  Side=Right
  Redacted_8840 : PMIOPort  Port=5  Side=Right
  connections:
  Redacted_8840/RConn1 -- Redacted_5818/RConn1
  Open Circuit/LConn1 -- Redacted_8974/RConn1
  Redacted_9727/RConn1 -- Redacted_9930/RConn1

== system Electrical_System_2018b_obfs/Redacted_1221/Redacted_7996/Redacted_9242/Redacted_38/Redacted_8107/Redacted_8444/Positive_Neutral ==
  Open Circuit : fl_lib/Electrical/Electrical Elements/Open Circuit  v_specify=off  v_priority=None  v=0 V  v_nominal_specify=off  v_nominal_unit=V  v_nominal_value=1
      settings: SourceProductName=Simscape  SourceProductBaseCode=SS
  Redacted_8974 : PMIOPort  Side=Left
  Redacted_9727 : PMIOPort  Port=2  Side=Left
  Redacted_5818 : PMIOPort  Port=3  Side=Left
  Redacted_9930 : PMIOPort  Port=4  Side=Right
  Redacted_8840 : PMIOPort  Port=5  Side=Right
  connections:
  Open Circuit/LConn1 -- Redacted_5818/RConn1
  Redacted_9930/RConn1 -- Redacted_8974/RConn1
  Redacted_9727/RConn1 -- Redacted_8840/RConn1

== system Electrical_System_2018b_obfs/Redacted_1221/Redacted_7996/Redacted_9242/Redacted_38/Redacted_8107/Redacted_8444/Redacted_3917 ==
  Redacted_1857 : fl_lib/Electrical/Electrical Elements/Open Circuit  v_specify=off  v_priority=None  v=xcvpklmsqm V  v_nominal_specify=off  v_nominal_unit=V  v_nominal_value=rzgrfophqu
      settings: SourceProductName=Simscape  SourceProductBaseCode=SS
  Redacted_8974 : PMIOPort  Side=Left
  Redacted_9727 : PMIOPort  Port=2  Side=Left
  Redacted_5818 : PMIOPort  Port=3  Side=Left
  Redacted_9930 : PMIOPort  Port=4  Side=Right
  Redacted_8840 : PMIOPort  Port=5  Side=Right
  connections:
  Redacted_1857/LConn1 -- Redacted_9727/RConn1
  Redacted_9930/RConn1 -- Redacted_8974/RConn1
  Redacted_8840/RConn1 -- Redacted_5818/RConn1
